simulink model "FM_Bistatic_Radar_Full"  (R2025a)
settings: Solver=VariableStepAuto  StartTime=0.0  StopTime=10.0  RelTol=1e-3
libraries: dspadpt3 x1, commanabbnd3 x1
(part 1 of 3)
settings Model: Creator=leifefrancisco  LastModifiedBy=leifefrancisco

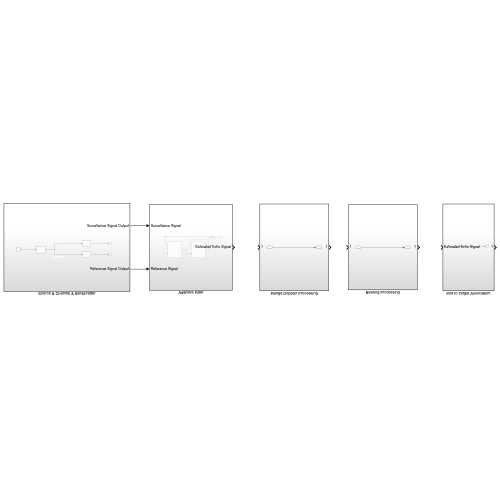
[thumbnail: Simulink's stored preview of the top-level diagram]
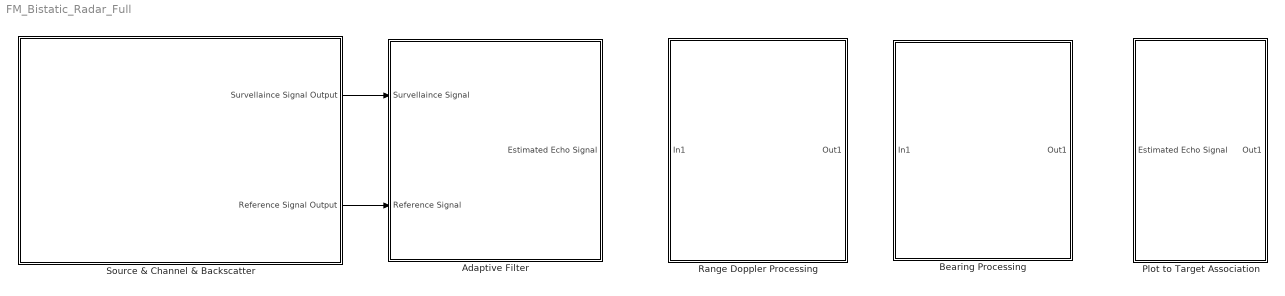
== system FM_Bistatic_Radar_Full ==
  Adaptive Filter : Subsystem
  Bearing Processing : Subsystem
  Plot to Target Association : Subsystem
  Range Doppler Processing : Subsystem
  Source & Channel & Backscatter : Subsystem
  wires:
  Source & Channel & Backscatter/1(Survellaince Signal Output) -> Adaptive Filter/1(Survellaince Signal)
  Source & Channel & Backscatter/2(Reference Signal Output) -> Adaptive Filter/2(Reference Signal)

== system FM_Bistatic_Radar_Full/Adaptive Filter ==
  Survellaince Signal : Inport
  Reference Signal : Inport  Port=2
  Gradiant Adaptive Lattice : Subsystem
  Subtract : Sum  Inputs=+-
  Tapped Delay Line : Subsystem
  Estimated Echo Signal : Outport
  wires:
  Reference Signal/1 -> Gradiant Adaptive Lattice/2(Backwards Propogation Error)
  Survellaince Signal/1 -> Gradiant Adaptive Lattice/1(Forward Propogation Error), Subtract/1
  Gradiant Adaptive Lattice/1(Backards Propogation Error Output) -> Tapped Delay Line/2(Backwards Propogation Errors)
  Tapped Delay Line/1(Error Signal) -> Subtract/2
  Subtract/1 -> Tapped Delay Line/1(Estimated Echo Signal), Estimated Echo Signal/1

== system FM_Bistatic_Radar_Full/Bearing Processing ==
  In1 : Inport
  Out1 : Outport
  wires:
  In1/1 -> Out1/1

== system FM_Bistatic_Radar_Full/Plot to Target Association ==
  Estimated Echo Signal : Inport
  Out1 : Outport
  wires:
  Estimated Echo Signal/1 -> Out1/1

== system FM_Bistatic_Radar_Full/Range Doppler Processing ==
  In1 : Inport
  Out1 : Outport
  wires:
  In1/1 -> Out1/1

== system FM_Bistatic_Radar_Full/Source & Channel & Backscatter ==
  note: Put that function that you made in your matlab code
  note: Survellaince Signal
  note: Reference Signal
  FM Modulator Baseband : commanabbnd3/FM Modulator Baseband  FrequencyDeviation=75e3  SimulateUsing=Code generation
  MATLAB Function : MATLAB Function  TreatAsAtomicUnit=on
  MATLAB Function1 : MATLAB Function  TreatAsAtomicUnit=on
  Sine Wave : Sin  Frequency=2*pi*200*1000  SampleTime=1/10000
  Survellaince Signal Output : Outport
  Reference Signal Output : Outport  Port=2
  wires:
  MATLAB Function/1(y) -> Survellaince Signal Output/1
  MATLAB Function1/1(y) -> Reference Signal Output/1
  Sine Wave/1 -> FM Modulator Baseband/1
  FM Modulator Baseband/1 -> MATLAB Function1/1(u), MATLAB Function/1(u)

== system FM_Bistatic_Radar_Full/Adaptive Filter/Gradiant Adaptive Lattice ==
  Forward Propogation Error : Inport
  Backwards Propogation Error : Inport  Port=2
  50-Stage Lattice Predictor : Subsystem
  Sum of Elements : Sum  Inputs=++++++++++
  Backards Propogation Error Output : Outport
  wires:
  Forward Propogation Error/1 -> 50-Stage Lattice Predictor/1(Forward Prediction Error)
  Backwards Propogation Error/1 -> 50-Stage Lattice Predictor/2(Backward Prediction Error)
  50-Stage Lattice Predictor/1(Backwards Propogation Error1) -> Sum of Elements/1
  50-Stage Lattice Predictor/2(Backwards Propogation Error2) -> Sum of Elements/2
  50-Stage Lattice Predictor/3(Backwards Propogation Error3) -> Sum of Elements/3
  50-Stage Lattice Predictor/4(Backwards Propogation Error4) -> Sum of Elements/4
  50-Stage Lattice Predictor/5(Backwards Propogation Error5) -> Sum of Elements/5
  50-Stage Lattice Predictor/6(Backwards Propogation Error6) -> Sum of Elements/6
  50-Stage Lattice Predictor/7(Backwards Propogation Error7) -> Sum of Elements/7
  50-Stage Lattice Predictor/8(Backwards Propogation Error8) -> Sum of Elements/8
  50-Stage Lattice Predictor/9(Backwards Propogation Error9) -> Sum of Elements/9
  50-Stage Lattice Predictor/10(Backwards Propogation Error10) -> Sum of Elements/10
  Sum of Elements/1 -> Backards Propogation Error Output/1

== system FM_Bistatic_Radar_Full/Adaptive Filter/Tapped Delay Line ==
  Estimated Echo Signal : Inport
  Backwards Propogation Errors : Inport  Port=2
  LMS Filter : dspadpt3/LMS Filter  Algo=LMS  L=32  stepflag=Dialog  mu=0.1  leakage=1.0  ic=0  Adapt=off  resetflag=None  weights=on  addnparflag=off  roundingMode=Floor  overflowMode=off  secondCoeffMode=Binary point scaling  secondCoeffWordLength=2  secondCoeffFracLength=15  prodOutput2Mode=Binary point scaling  prodOutput2FracLength=20  prodOutput3Mode=Binary point scaling  prodOutput3FracLength=20  prodOutput4Mode=Binary point scaling  prodOutput4FracLength=20  quotientMode=Binary point scaling  quotientFracLength=20  accum2Mode=Binary point scaling  accum2FracLength=20
      settings: LibrarySourceBlock=dsphdlsupportfiltering/LMS Filter
  Scope : Scope
  Scope1 : Scope
  Error Signal : Outport
  wires:
  Estimated Echo Signal/1 -> LMS Filter/1
  Backwards Propogation Errors/1 -> LMS Filter/2
  LMS Filter/2 -> Error Signal/1
  LMS Filter/1 -> Scope/1
  LMS Filter/3 -> Scope1/1

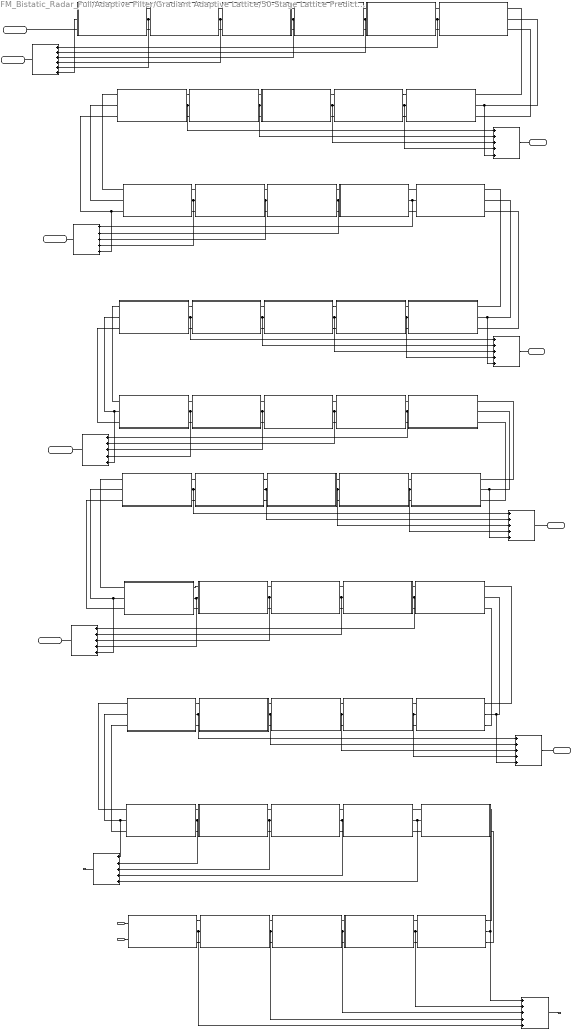
== system FM_Bistatic_Radar_Full/Adaptive Filter/Gradiant Adaptive Lattice/50-Stage Lattice Predictor ==
  Forward Prediction Error : Inport
  Backward Prediction Error : Inport  Port=2
  Stage 1 : Subsystem
  Stage 10 : Subsystem
  Stage 11 : Subsystem
  Stage 12 : Subsystem
  Stage 13 : Subsystem
  Stage 14 : Subsystem
  Stage 15 : Subsystem
  Stage 16 : Subsystem
  Stage 17 : Subsystem
  Stage 18 : Subsystem
  Stage 19 : Subsystem
  Stage 2 : Subsystem
  Stage 20 : Subsystem
  Stage 21 : Subsystem
  Stage 22 : Subsystem
  Stage 23 : Subsystem
  Stage 24 : Subsystem
  Stage 25 : Subsystem
  Stage 26 : Subsystem
  Stage 27 : Subsystem
  Stage 28 : Subsystem
  Stage 29 : Subsystem
  Stage 3 : Subsystem
  Stage 30 : Subsystem
  Stage 31 : Subsystem
  Stage 32 : Subsystem
  Stage 33 : Subsystem
  Stage 34 : Subsystem
  Stage 35 : Subsystem
  Stage 36 : Subsystem
  Stage 37 : Subsystem
  Stage 38 : Subsystem
  Stage 39 : Subsystem
  Stage 4 : Subsystem
  Stage 40 : Subsystem
  Stage 41 : Subsystem
  Stage 42 : Subsystem
  Stage 43 : Subsystem
  Stage 44 : Subsystem
  Stage 45 : Subsystem
  Stage 46 : Subsystem
  Stage 47 : Subsystem
  Stage 48 : Subsystem
  Stage 49 : Subsystem
  Stage 5 : Subsystem
  Stage 50 : Subsystem
  Stage 51 : Subsystem
  Stage 6 : Subsystem
  Stage 7 : Subsystem
  Stage 8 : Subsystem
  Stage 9 : Subsystem
  Sum of Elements{1..9} (9 alike) : Sum  Inputs=+++++
  Sum of Elements10 : Sum  Inputs=++++++
  Backwards Propogation Error1 : Outport
  Backwards Propogation Error2 : Outport  Port=2
  Backwards Propogation Error3 : Outport  Port=3
  Backwards Propogation Error4 : Outport  Port=4
  Backwards Propogation Error5 : Outport  Port=5
  Backwards Propogation Error6 : Outport  Port=6
  Backwards Propogation Error7 : Outport  Port=7
  Backwards Propogation Error8 : Outport  Port=8
  Backwards Propogation Error9 : Outport  Port=9
  Backwards Propogation Error10 : Outport  Port=10
  K Final : Outport  Port=11
  wires:
  Stage 9/2(Backward Prediction Error Output) -> Sum of Elements2/2, Stage 10/2(Backward Prediction Error)
  Backward Prediction Error/1 -> Stage 1/2(Backward Prediction Error)
  Stage 50/1(Forward Prediction Error Output) -> Stage 51/1(Forward Prediction Error)
  Stage 29/3(K) -> Stage 30/3(K Input)
  Stage 21/3(K) -> Stage 22/3(K Input)
  Stage 36/3(K) -> Stage 37/3(K Input)
  Stage 27/3(K) -> Stage 28/3(K Input)
  Stage 15/3(K) -> Stage 16/3(K Input)
  Stage 20/3(K) -> Stage 21/3(K Input)
  Stage 49/1(Forward Prediction Error Output) -> Stage 50/1(Forward Prediction Error)
  Stage 47/3(K) -> Stage 48/3(K Input)
  Stage 20/2(Backward Prediction Error Output) -> Sum of Elements6/3, Stage 21/2(Backward Prediction Error)
  Stage 46/1(Forward Prediction Error Output) -> Stage 47/1(Forward Prediction Error)
  Stage 18/1(Forward Prediction Error Output) -> Stage 19/1(Forward Prediction Error)
  Stage 5/3(K) -> Stage 6/3(K Input)
  Stage 46/3(K) -> Stage 47/3(K Input)
  Stage 17/2(Backward Prediction Error Output) -> Sum of Elements4/2, Stage 26/2(Backward Prediction Error)
  Stage 50/2(Backward Prediction Error Output) -> Sum of Elements10/5, Stage 51/2(Backward Prediction Error)
  Stage 25/3(K) -> Stage 34/3(K Input)
  Forward Prediction Error/1 -> Stage 1/1(Forward Prediction Error)
  Stage 38/3(K) -> Stage 39/3(K Input)
  Stage 11/2(Backward Prediction Error Output) -> Sum of Elements3/1, Stage 12/2(Backward Prediction Error)
  Stage 2/3(K) -> Stage 3/3(K Input)
  Stage 24/2(Backward Prediction Error Output) -> Sum of Elements7/2, Stage 25/2(Backward Prediction Error)
  Stage 7/2(Backward Prediction Error Output) -> Sum of Elements2/4, Stage 8/2(Backward Prediction Error)
  Stage 18/2(Backward Prediction Error Output) -> Sum of Elements6/1, Stage 19/2(Backward Prediction Error)
  Stage 37/2(Backward Prediction Error Output) -> Sum of Elements8/2, Stage 38/2(Backward Prediction Error)
  Stage 32/2(Backward Prediction Error Output) -> Sum of Elements5/4, Stage 33/2(Backward Prediction Error)
  Stage 48/2(Backward Prediction Error Output) -> Sum of Elements10/3, Stage 49/2(Backward Prediction Error)
  Stage 49/3(K) -> Stage 50/3(K Input)
  Stage 30/1(Forward Prediction Error Output) -> Stage 31/1(Forward Prediction Error)
  Stage 21/2(Backward Prediction Error Output) -> Sum of Elements6/4, Stage 22/2(Backward Prediction Error)
  Stage 38/1(Forward Prediction Error Output) -> Stage 39/1(Forward Prediction Error)
  Stage 39/2(Backward Prediction Error Output) -> Sum of Elements8/4, Stage 40/2(Backward Prediction Error)
  Stage 21/1(Forward Prediction Error Output) -> Stage 22/1(Forward Prediction Error)
  Stage 36/2(Backward Prediction Error Output) -> Sum of Elements8/1, Stage 37/2(Backward Prediction Error)
  Stage 34/3(K) -> Stage 35/3(K Input)
  Stage 29/1(Forward Prediction Error Output) -> Stage 30/1(Forward Prediction Error)
  Stage 48/1(Forward Prediction Error Output) -> Stage 49/1(Forward Prediction Error)
  Stage 39/3(K) -> Stage 40/3(K Input)
  Stage 3/3(K) -> Stage 4/3(K Input)
  Stage 14/3(K) -> Stage 15/3(K Input)
  Stage 25/1(Forward Prediction Error Output) -> Stage 34/1(Forward Prediction Error)
  Stage 19/3(K) -> Stage 20/3(K Input)
  Stage 24/1(Forward Prediction Error Output) -> Stage 25/1(Forward Prediction Error)
  Stage 9/1(Forward Prediction Error Output) -> Stage 10/1(Forward Prediction Error)
  Stage 24/3(K) -> Stage 25/3(K Input)
  Stage 17/3(K) -> Stage 26/3(K Input)
  Stage 29/2(Backward Prediction Error Output) -> Sum of Elements5/1, Stage 30/2(Backward Prediction Error)
  Stage 7/1(Forward Prediction Error Output) -> Stage 8/1(Forward Prediction Error)
  Stage 34/2(Backward Prediction Error Output) -> Sum of Elements7/4, Stage 35/2(Backward Prediction Error)
  Stage 19/1(Forward Prediction Error Output) -> Stage 20/1(Forward Prediction Error)
  Stage 1/1(Forward Prediction Error Output) -> Stage 2/1(Forward Prediction Error)
  Stage 23/3(K) -> Stage 24/3(K Input)
  Stage 23/2(Backward Prediction Error Output) -> Sum of Elements7/1, Stage 24/2(Backward Prediction Error)
  Stage 37/3(K) -> Stage 38/3(K Input)
  Stage 20/1(Forward Prediction Error Output) -> Stage 21/1(Forward Prediction Error)
  Stage 19/2(Backward Prediction Error Output) -> Sum of Elements6/2, Stage 20/2(Backward Prediction Error)
  Stage 34/1(Forward Prediction Error Output) -> Stage 35/1(Forward Prediction Error)
  Stage 23/1(Forward Prediction Error Output) -> Stage 24/1(Forward Prediction Error)
  Stage 6/1(Forward Prediction Error Output) -> Stage 7/1(Forward Prediction Error)
  Stage 4/3(K) -> Stage 5/3(K Input)
  Stage 12/1(Forward Prediction Error Output) -> Stage 13/1(Forward Prediction Error)
  Stage 32/1(Forward Prediction Error Output) -> Stage 33/1(Forward Prediction Error)
  Stage 32/3(K) -> Stage 33/3(K Input)
  Stage 39/1(Forward Prediction Error Output) -> Stage 40/1(Forward Prediction Error)
  Stage 1/3(K) -> Stage 2/3(K Input)
  Stage 8/1(Forward Prediction Error Output) -> Stage 9/1(Forward Prediction Error)
  Stage 26/2(Backward Prediction Error Output) -> Sum of Elements4/3, Stage 27/2(Backward Prediction Error)
  Stage 27/2(Backward Prediction Error Output) -> Sum of Elements4/4, Stage 28/2(Backward Prediction Error)
  Stage 25/2(Backward Prediction Error Output) -> Sum of Elements7/3, Stage 34/2(Backward Prediction Error)
  Stage 6/3(K) -> Stage 7/3(K Input)
  Stage 27/1(Forward Prediction Error Output) -> Stage 28/1(Forward Prediction Error)
  Stage 30/3(K) -> Stage 31/3(K Input)
  Stage 3/2(Backward Prediction Error Output) -> Sum of Elements1/3, Stage 4/2(Backward Prediction Error)
  Stage 31/3(K) -> Stage 32/3(K Input)
  Stage 47/1(Forward Prediction Error Output) -> Stage 48/1(Forward Prediction Error)
  Stage 49/2(Backward Prediction Error Output) -> Sum of Elements10/4, Stage 50/2(Backward Prediction Error)
  Stage 46/2(Backward Prediction Error Output) -> Sum of Elements10/1, Stage 47/2(Backward Prediction Error)
  Stage 26/3(K) -> Stage 27/3(K Input)
  Stage 11/1(Forward Prediction Error Output) -> Stage 12/1(Forward Prediction Error)
  Stage 31/2(Backward Prediction Error Output) -> Sum of Elements5/3, Stage 32/2(Backward Prediction Error)
  Stage 50/3(K) -> Stage 51/3(K Input)
  Stage 31/1(Forward Prediction Error Output) -> Stage 32/1(Forward Prediction Error)
  Stage 26/1(Forward Prediction Error Output) -> Stage 27/1(Forward Prediction Error)
  Stage 48/3(K) -> Stage 49/3(K Input)
  Stage 37/1(Forward Prediction Error Output) -> Stage 38/1(Forward Prediction Error)
  Stage 4/2(Backward Prediction Error Output) -> Sum of Elements1/2, Stage 5/2(Backward Prediction Error)
  Stage 2/1(Forward Prediction Error Output) -> Stage 3/1(Forward Prediction Error)
  Stage 17/1(Forward Prediction Error Output) -> Stage 26/1(Forward Prediction Error)
  Stage 16/2(Backward Prediction Error Output) -> Sum of Elements4/1, Stage 17/2(Backward Prediction Error)
  Stage 15/2(Backward Prediction Error Output) -> Sum of Elements3/5, Stage 16/2(Backward Prediction Error)
  Stage 18/3(K) -> Stage 19/3(K Input)
  Stage 14/1(Forward Prediction Error Output) -> Stage 15/1(Forward Prediction Error)
  Stage 12/2(Backward Prediction Error Output) -> Sum of Elements3/2, Stage 13/2(Backward Prediction Error)
  Stage 38/2(Backward Prediction Error Output) -> Sum of Elements8/3, Stage 39/2(Backward Prediction Error)
  Stage 8/2(Backward Prediction Error Output) -> Sum of Elements2/3, Stage 9/2(Backward Prediction Error)
  Stage 13/1(Forward Prediction Error Output) -> Stage 14/1(Forward Prediction Error)
  Stage 16/1(Forward Prediction Error Output) -> Stage 17/1(Forward Prediction Error)
  Stage 5/1(Forward Prediction Error Output) -> Stage 6/1(Forward Prediction Error)
  Stage 14/2(Backward Prediction Error Output) -> Sum of Elements3/4, Stage 15/2(Backward Prediction Error)
  Stage 6/2(Backward Prediction Error Output) -> Sum of Elements2/5, Stage 7/2(Backward Prediction Error)
  Stage 12/3(K) -> Stage 13/3(K Input)
  Stage 16/3(K) -> Stage 17/3(K Input)
  Stage 15/1(Forward Prediction Error Output) -> Stage 16/1(Forward Prediction Error)
  Stage 13/2(Backward Prediction Error Output) -> Sum of Elements3/3, Stage 14/2(Backward Prediction Error)
  Stage 11/3(K) -> Stage 12/3(K Input)
  Stage 4/1(Forward Prediction Error Output) -> Stage 5/1(Forward Prediction Error)
  Stage 5/2(Backward Prediction Error Output) -> Sum of Elements1/1, Stage 6/2(Backward Prediction Error)
  Stage 9/3(K) -> Stage 10/3(K Input)
  Stage 8/3(K) -> Stage 9/3(K Input)
  Stage 13/3(K) -> Stage 14/3(K Input)
  Stage 7/3(K) -> Stage 8/3(K Input)
  Stage 36/1(Forward Prediction Error Output) -> Stage 37/1(Forward Prediction Error)
  Stage 3/1(Forward Prediction Error Output) -> Stage 4/1(Forward Prediction Error)
  Stage 47/2(Backward Prediction Error Output) -> Sum of Elements10/2, Stage 48/2(Backward Prediction Error)
  Stage 30/2(Backward Prediction Error Output) -> Sum of Elements5/2, Stage 31/2(Backward Prediction Error)
  Stage 1/2(Backward Prediction Error Output) -> Sum of Elements1/5, Stage 2/2(Backward Prediction Error)
  Stage 10/3(K) -> Stage 11/3(K Input)
  Stage 10/2(Backward Prediction Error Output) -> Sum of Elements2/1, Stage 11/2(Backward Prediction Error)
  Stage 10/1(Forward Prediction Error Output) -> Stage 11/1(Forward Prediction Error)
  Stage 28/3(K) -> Stage 29/3(K Input)
  Stage 28/2(Backward Prediction Error Output) -> Sum of Elements4/5, Stage 29/2(Backward Prediction Error)
  Stage 28/1(Forward Prediction Error Output) -> Stage 29/1(Forward Prediction Error)
  Stage 33/3(K) -> Stage 18/3(K Input)
  Stage 33/2(Backward Prediction Error Output) -> Sum of Elements5/5, Stage 18/2(Backward Prediction Error)
  Stage 33/1(Forward Prediction Error Output) -> Stage 18/1(Forward Prediction Error)
  Stage 22/3(K) -> Stage 23/3(K Input)
  Stage 22/2(Backward Prediction Error Output) -> Sum of Elements6/5, Stage 23/2(Backward Prediction Error)
  Stage 22/1(Forward Prediction Error Output) -> Stage 23/1(Forward Prediction Error)
  Stage 35/3(K) -> Stage 36/3(K Input)
  Stage 35/2(Backward Prediction Error Output) -> Sum of Elements7/5, Stage 36/2(Backward Prediction Error)
  Stage 35/1(Forward Prediction Error Output) -> Stage 36/1(Forward Prediction Error)
  Stage 40/2(Backward Prediction Error Output) -> Stage 41/2(Backward Prediction Error)
  Stage 40/1(Forward Prediction Error Output) -> Stage 41/1(Forward Prediction Error)
  Stage 41/1(Forward Prediction Error Output) -> Stage 42/1(Forward Prediction Error)
  Stage 41/2(Backward Prediction Error Output) -> Sum of Elements9/1, Stage 42/2(Backward Prediction Error)
  Stage 41/3(K) -> Stage 42/3(K Input)
  Stage 42/1(Forward Prediction Error Output) -> Stage 43/1(Forward Prediction Error)
  Stage 42/2(Backward Prediction Error Output) -> Sum of Elements9/2, Stage 43/2(Backward Prediction Error)
  Stage 42/3(K) -> Stage 43/3(K Input)
  Stage 43/1(Forward Prediction Error Output) -> Stage 44/1(Forward Prediction Error)
  Stage 43/2(Backward Prediction Error Output) -> Sum of Elements9/3, Stage 44/2(Backward Prediction Error)
  Stage 43/3(K) -> Stage 44/3(K Input)
  Stage 44/1(Forward Prediction Error Output) -> Stage 45/1(Forward Prediction Error)
  Stage 44/2(Backward Prediction Error Output) -> Sum of Elements9/4, Stage 45/2(Backward Prediction Error)
  Stage 44/3(K) -> Stage 45/3(K Input)
  Stage 45/3(K) -> Stage 46/3(K Input)
  Stage 45/2(Backward Prediction Error Output) -> Sum of Elements9/5, Stage 46/2(Backward Prediction Error)
  Stage 45/1(Forward Prediction Error Output) -> Stage 46/1(Forward Prediction Error)
  Stage 40/3(K) -> Stage 41/3(K Input), Sum of Elements8/5
  Stage 2/2(Backward Prediction Error Output) -> Sum of Elements1/4, Stage 3/2(Backward Prediction Error)
  Sum of Elements1/1 -> Backwards Propogation Error1/1
  Sum of Elements2/1 -> Backwards Propogation Error2/1
  Stage 51/2(Backward Prediction Error Output) -> Sum of Elements10/6
  Sum of Elements10/1 -> Backwards Propogation Error10/1
  Sum of Elements8/1 -> Backwards Propogation Error8/1
  Sum of Elements6/1 -> Backwards Propogation Error6/1
  Sum of Elements4/1 -> Backwards Propogation Error4/1
  Sum of Elements3/1 -> Backwards Propogation Error3/1
  Sum of Elements5/1 -> Backwards Propogation Error5/1
  Sum of Elements7/1 -> Backwards Propogation Error7/1
  Sum of Elements9/1 -> Backwards Propogation Error9/1
  Stage 51/3(K) -> K Final/1

== system FM_Bistatic_Radar_Full/Adaptive Filter/Gradiant Adaptive Lattice/50-Stage Lattice Predictor/Stage 1 ==
  note: K Update
  Forward Prediction Error : Inport
  Backward Prediction Error : Inport  Port=2
  Delay : Delay  DelayLength=1  InitialCondition=0
  K Update Equation : Subsystem
  Sum : Sum  Inputs=|++
  Sum1 : Sum  Inputs=|++
  Forward Prediction Error Output : Outport
  Backward Prediction Error Output : Outport  Port=2
  K : Outport  Port=3
  wires:
  Sum1/1 -> Backward Prediction Error Output/1
  Delay/1 -> Sum1/2, K Update Equation/2(B I/P)
  Sum/1 -> Forward Prediction Error Output/1
  K Update Equation/2(K) -> K/1, Sum1/1
  K Update Equation/1(*K (K conjugate)) -> Sum/2
  Backward Prediction Error/1 -> Delay/1
  Forward Prediction Error/1 -> Sum/1, K Update Equation/1(F I/P)

== system FM_Bistatic_Radar_Full/Adaptive Filter/Gradiant Adaptive Lattice/50-Stage Lattice Predictor/Stage 10 ==
  note: K Update
  Forward Prediction Error : Inport
  Backward Prediction Error : Inport  Port=2
  K Input : Inport  Port=3
  Delay : Delay  DelayLength=1  InitialCondition=0
  K Update Equation : Subsystem
  Sum : Sum  Inputs=|++
  Sum1 : Sum  Inputs=|++
  Forward Prediction Error Output : Outport
  Backward Prediction Error Output : Outport  Port=2
  K : Outport  Port=3
  wires:
  Sum1/1 -> Backward Prediction Error Output/1
  Delay/1 -> Sum1/2, K Update Equation/2(B I/P)
  Sum/1 -> Forward Prediction Error Output/1
  K Update Equation/2(K) -> K/1, Sum1/1
  K Update Equation/1(*K (K conjugate)) -> Sum/2
  Backward Prediction Error/1 -> Delay/1
  Forward Prediction Error/1 -> Sum/1, K Update Equation/1(F I/P)
  K Input/1 -> K Update Equation/3(K I/P)

== system FM_Bistatic_Radar_Full/Adaptive Filter/Gradiant Adaptive Lattice/50-Stage Lattice Predictor/Stage 11 ==
  note: K Update
  Forward Prediction Error : Inport
  Backward Prediction Error : Inport  Port=2
  K Input : Inport  Port=3
  Delay : Delay  DelayLength=1  InitialCondition=0
  K Update Equation : Subsystem
  Sum : Sum  Inputs=|++
  Sum1 : Sum  Inputs=|++
  Forward Prediction Error Output : Outport
  Backward Prediction Error Output : Outport  Port=2
  K : Outport  Port=3
  wires:
  Sum1/1 -> Backward Prediction Error Output/1
  Delay/1 -> Sum1/2, K Update Equation/2(B I/P)
  Sum/1 -> Forward Prediction Error Output/1
  K Update Equation/2(K) -> K/1, Sum1/1
  K Update Equation/1(*K (K conjugate)) -> Sum/2
  Backward Prediction Error/1 -> Delay/1
  Forward Prediction Error/1 -> Sum/1, K Update Equation/1(F I/P)
  K Input/1 -> K Update Equation/3(K I/P)

== system FM_Bistatic_Radar_Full/Adaptive Filter/Gradiant Adaptive Lattice/50-Stage Lattice Predictor/Stage 12 ==
  note: K Update
  Forward Prediction Error : Inport
  Backward Prediction Error : Inport  Port=2
  K Input : Inport  Port=3
  Delay : Delay  DelayLength=1  InitialCondition=0
  K Update Equation : Subsystem
  Sum : Sum  Inputs=|++
  Sum1 : Sum  Inputs=|++
  Forward Prediction Error Output : Outport
  Backward Prediction Error Output : Outport  Port=2
  K : Outport  Port=3
  wires:
  Sum1/1 -> Backward Prediction Error Output/1
  Delay/1 -> Sum1/2, K Update Equation/2(B I/P)
  Sum/1 -> Forward Prediction Error Output/1
  K Update Equation/2(K) -> K/1, Sum1/1
  K Update Equation/1(*K (K conjugate)) -> Sum/2
  Backward Prediction Error/1 -> Delay/1
  Forward Prediction Error/1 -> Sum/1, K Update Equation/1(F I/P)
  K Input/1 -> K Update Equation/3(K I/P)

== system FM_Bistatic_Radar_Full/Adaptive Filter/Gradiant Adaptive Lattice/50-Stage Lattice Predictor/Stage 13 ==
  note: K Update
  Forward Prediction Error : Inport
  Backward Prediction Error : Inport  Port=2
  K Input : Inport  Port=3
  Delay : Delay  DelayLength=1  InitialCondition=0
  K Update Equation : Subsystem
  Sum : Sum  Inputs=|++
  Sum1 : Sum  Inputs=|++
  Forward Prediction Error Output : Outport
  Backward Prediction Error Output : Outport  Port=2
  K : Outport  Port=3
  wires:
  Sum1/1 -> Backward Prediction Error Output/1
  Delay/1 -> Sum1/2, K Update Equation/2(B I/P)
  Sum/1 -> Forward Prediction Error Output/1
  K Update Equation/2(K) -> K/1, Sum1/1
  K Update Equation/1(*K (K conjugate)) -> Sum/2
  Backward Prediction Error/1 -> Delay/1
  Forward Prediction Error/1 -> Sum/1, K Update Equation/1(F I/P)
  K Input/1 -> K Update Equation/3(K I/P)

== system FM_Bistatic_Radar_Full/Adaptive Filter/Gradiant Adaptive Lattice/50-Stage Lattice Predictor/Stage 14 ==
  note: K Update
  Forward Prediction Error : Inport
  Backward Prediction Error : Inport  Port=2
  K Input : Inport  Port=3
  Delay : Delay  DelayLength=1  InitialCondition=0
  K Update Equation : Subsystem
  Sum : Sum  Inputs=|++
  Sum1 : Sum  Inputs=|++
  Forward Prediction Error Output : Outport
  Backward Prediction Error Output : Outport  Port=2
  K : Outport  Port=3
  wires:
  Sum1/1 -> Backward Prediction Error Output/1
  Delay/1 -> Sum1/2, K Update Equation/2(B I/P)
  Sum/1 -> Forward Prediction Error Output/1
  K Update Equation/2(K) -> K/1, Sum1/1
  K Update Equation/1(*K (K conjugate)) -> Sum/2
  Backward Prediction Error/1 -> Delay/1
  Forward Prediction Error/1 -> Sum/1, K Update Equation/1(F I/P)
  K Input/1 -> K Update Equation/3(K I/P)

== system FM_Bistatic_Radar_Full/Adaptive Filter/Gradiant Adaptive Lattice/50-Stage Lattice Predictor/Stage 15 ==
  note: K Update
  Forward Prediction Error : Inport
  Backward Prediction Error : Inport  Port=2
  K Input : Inport  Port=3
  Delay : Delay  DelayLength=1  InitialCondition=0
  K Update Equation : Subsystem
  Sum : Sum  Inputs=|++
  Sum1 : Sum  Inputs=|++
  Forward Prediction Error Output : Outport
  Backward Prediction Error Output : Outport  Port=2
  K : Outport  Port=3
  wires:
  Sum1/1 -> Backward Prediction Error Output/1
  Delay/1 -> Sum1/2, K Update Equation/2(B I/P)
  Sum/1 -> Forward Prediction Error Output/1
  K Update Equation/2(K) -> K/1, Sum1/1
  K Update Equation/1(*K (K conjugate)) -> Sum/2
  Backward Prediction Error/1 -> Delay/1
  Forward Prediction Error/1 -> Sum/1, K Update Equation/1(F I/P)
  K Input/1 -> K Update Equation/3(K I/P)

== system FM_Bistatic_Radar_Full/Adaptive Filter/Gradiant Adaptive Lattice/50-Stage Lattice Predictor/Stage 16 ==
  note: K Update
  Forward Prediction Error : Inport
  Backward Prediction Error : Inport  Port=2
  K Input : Inport  Port=3
  Delay : Delay  DelayLength=1  InitialCondition=0
  K Update Equation : Subsystem
  Sum : Sum  Inputs=|++
  Sum1 : Sum  Inputs=|++
  Forward Prediction Error Output : Outport
  Backward Prediction Error Output : Outport  Port=2
  K : Outport  Port=3
  wires:
  Sum1/1 -> Backward Prediction Error Output/1
  Delay/1 -> Sum1/2, K Update Equation/2(B I/P)
  Sum/1 -> Forward Prediction Error Output/1
  K Update Equation/2(K) -> K/1, Sum1/1
  K Update Equation/1(*K (K conjugate)) -> Sum/2
  Backward Prediction Error/1 -> Delay/1
  Forward Prediction Error/1 -> Sum/1, K Update Equation/1(F I/P)
  K Input/1 -> K Update Equation/3(K I/P)

== system FM_Bistatic_Radar_Full/Adaptive Filter/Gradiant Adaptive Lattice/50-Stage Lattice Predictor/Stage 17 ==
  note: K Update
  Forward Prediction Error : Inport
  Backward Prediction Error : Inport  Port=2
  K Input : Inport  Port=3
  Delay : Delay  DelayLength=1  InitialCondition=0
  K Update Equation : Subsystem
  Sum : Sum  Inputs=|++
  Sum1 : Sum  Inputs=|++
  Forward Prediction Error Output : Outport
  Backward Prediction Error Output : Outport  Port=2
  K : Outport  Port=3
  wires:
  Sum1/1 -> Backward Prediction Error Output/1
  Delay/1 -> Sum1/2, K Update Equation/2(B I/P)
  Sum/1 -> Forward Prediction Error Output/1
  K Update Equation/2(K) -> K/1, Sum1/1
  K Update Equation/1(*K (K conjugate)) -> Sum/2
  Backward Prediction Error/1 -> Delay/1
  Forward Prediction Error/1 -> Sum/1, K Update Equation/1(F I/P)
  K Input/1 -> K Update Equation/3(K I/P)

== system FM_Bistatic_Radar_Full/Adaptive Filter/Gradiant Adaptive Lattice/50-Stage Lattice Predictor/Stage 18 ==
  note: K Update
  Forward Prediction Error : Inport
  Backward Prediction Error : Inport  Port=2
  K Input : Inport  Port=3
  Delay : Delay  DelayLength=1  InitialCondition=0
  K Update Equation : Subsystem
  Sum : Sum  Inputs=|++
  Sum1 : Sum  Inputs=|++
  Forward Prediction Error Output : Outport
  Backward Prediction Error Output : Outport  Port=2
  K : Outport  Port=3
  wires:
  Sum1/1 -> Backward Prediction Error Output/1
  Delay/1 -> Sum1/2, K Update Equation/2(B I/P)
  Sum/1 -> Forward Prediction Error Output/1
  K Update Equation/2(K) -> K/1, Sum1/1
  K Update Equation/1(*K (K conjugate)) -> Sum/2
  Backward Prediction Error/1 -> Delay/1
  Forward Prediction Error/1 -> Sum/1, K Update Equation/1(F I/P)
  K Input/1 -> K Update Equation/3(K I/P)

== system FM_Bistatic_Radar_Full/Adaptive Filter/Gradiant Adaptive Lattice/50-Stage Lattice Predictor/Stage 19 ==
  note: K Update
  Forward Prediction Error : Inport
  Backward Prediction Error : Inport  Port=2
  K Input : Inport  Port=3
  Delay : Delay  DelayLength=1  InitialCondition=0
  K Update Equation : Subsystem
  Sum : Sum  Inputs=|++
  Sum1 : Sum  Inputs=|++
  Forward Prediction Error Output : Outport
  Backward Prediction Error Output : Outport  Port=2
  K : Outport  Port=3
  wires:
  Sum1/1 -> Backward Prediction Error Output/1
  Delay/1 -> Sum1/2, K Update Equation/2(B I/P)
  Sum/1 -> Forward Prediction Error Output/1
  K Update Equation/2(K) -> K/1, Sum1/1
  K Update Equation/1(*K (K conjugate)) -> Sum/2
  Backward Prediction Error/1 -> Delay/1
  Forward Prediction Error/1 -> Sum/1, K Update Equation/1(F I/P)
  K Input/1 -> K Update Equation/3(K I/P)

== system FM_Bistatic_Radar_Full/Adaptive Filter/Gradiant Adaptive Lattice/50-Stage Lattice Predictor/Stage 2 ==
  note: K Update
  Forward Prediction Error : Inport
  Backward Prediction Error : Inport  Port=2
  K Input : Inport  Port=3
  Delay : Delay  DelayLength=1  InitialCondition=0
  K Update Equation : Subsystem
  Sum : Sum  Inputs=|++
  Sum1 : Sum  Inputs=|++
  Forward Prediction Error Output : Outport
  Backward Prediction Error Output : Outport  Port=2
  K : Outport  Port=3
  wires:
  Sum1/1 -> Backward Prediction Error Output/1
  Delay/1 -> Sum1/2, K Update Equation/2(B I/P)
  Sum/1 -> Forward Prediction Error Output/1
  K Update Equation/2(K) -> K/1, Sum1/1
  K Update Equation/1(*K (K conjugate)) -> Sum/2
  Backward Prediction Error/1 -> Delay/1
  Forward Prediction Error/1 -> Sum/1, K Update Equation/1(F I/P)
  K Input/1 -> K Update Equation/3(K I/P)

== system FM_Bistatic_Radar_Full/Adaptive Filter/Gradiant Adaptive Lattice/50-Stage Lattice Predictor/Stage 20 ==
  note: K Update
  Forward Prediction Error : Inport
  Backward Prediction Error : Inport  Port=2
  K Input : Inport  Port=3
  Delay : Delay  DelayLength=1  InitialCondition=0
  K Update Equation : Subsystem
  Sum : Sum  Inputs=|++
  Sum1 : Sum  Inputs=|++
  Forward Prediction Error Output : Outport
  Backward Prediction Error Output : Outport  Port=2
  K : Outport  Port=3
  wires:
  Sum1/1 -> Backward Prediction Error Output/1
  Delay/1 -> Sum1/2, K Update Equation/2(B I/P)
  Sum/1 -> Forward Prediction Error Output/1
  K Update Equation/2(K) -> K/1, Sum1/1
  K Update Equation/1(*K (K conjugate)) -> Sum/2
  Backward Prediction Error/1 -> Delay/1
  Forward Prediction Error/1 -> Sum/1, K Update Equation/1(F I/P)
  K Input/1 -> K Update Equation/3(K I/P)

== system FM_Bistatic_Radar_Full/Adaptive Filter/Gradiant Adaptive Lattice/50-Stage Lattice Predictor/Stage 21 ==
  note: K Update
  Forward Prediction Error : Inport
  Backward Prediction Error : Inport  Port=2
  K Input : Inport  Port=3
  Delay : Delay  DelayLength=1  InitialCondition=0
  K Update Equation : Subsystem
  Sum : Sum  Inputs=|++
  Sum1 : Sum  Inputs=|++
  Forward Prediction Error Output : Outport
  Backward Prediction Error Output : Outport  Port=2
  K : Outport  Port=3
  wires:
  Sum1/1 -> Backward Prediction Error Output/1
  Delay/1 -> Sum1/2, K Update Equation/2(B I/P)
  Sum/1 -> Forward Prediction Error Output/1
  K Update Equation/2(K) -> K/1, Sum1/1
  K Update Equation/1(*K (K conjugate)) -> Sum/2
  Backward Prediction Error/1 -> Delay/1
  Forward Prediction Error/1 -> Sum/1, K Update Equation/1(F I/P)
  K Input/1 -> K Update Equation/3(K I/P)

== system FM_Bistatic_Radar_Full/Adaptive Filter/Gradiant Adaptive Lattice/50-Stage Lattice Predictor/Stage 22 ==
  note: K Update
  Forward Prediction Error : Inport
  Backward Prediction Error : Inport  Port=2
  K Input : Inport  Port=3
  Delay : Delay  DelayLength=1  InitialCondition=0
  K Update Equation : Subsystem
  Sum : Sum  Inputs=|++
  Sum1 : Sum  Inputs=|++
  Forward Prediction Error Output : Outport
  Backward Prediction Error Output : Outport  Port=2
  K : Outport  Port=3
  wires:
  Sum1/1 -> Backward Prediction Error Output/1
  Delay/1 -> Sum1/2, K Update Equation/2(B I/P)
  Sum/1 -> Forward Prediction Error Output/1
  K Update Equation/2(K) -> K/1, Sum1/1
  K Update Equation/1(*K (K conjugate)) -> Sum/2
  Backward Prediction Error/1 -> Delay/1
  Forward Prediction Error/1 -> Sum/1, K Update Equation/1(F I/P)
  K Input/1 -> K Update Equation/3(K I/P)

== system FM_Bistatic_Radar_Full/Adaptive Filter/Gradiant Adaptive Lattice/50-Stage Lattice Predictor/Stage 23 ==
  note: K Update
  Forward Prediction Error : Inport
  Backward Prediction Error : Inport  Port=2
  K Input : Inport  Port=3
  Delay : Delay  DelayLength=1  InitialCondition=0
  K Update Equation : Subsystem
  Sum : Sum  Inputs=|++
  Sum1 : Sum  Inputs=|++
  Forward Prediction Error Output : Outport
  Backward Prediction Error Output : Outport  Port=2
  K : Outport  Port=3
  wires:
  Sum1/1 -> Backward Prediction Error Output/1
  Delay/1 -> Sum1/2, K Update Equation/2(B I/P)
  Sum/1 -> Forward Prediction Error Output/1
  K Update Equation/2(K) -> K/1, Sum1/1
  K Update Equation/1(*K (K conjugate)) -> Sum/2
  Backward Prediction Error/1 -> Delay/1
  Forward Prediction Error/1 -> Sum/1, K Update Equation/1(F I/P)
  K Input/1 -> K Update Equation/3(K I/P)

== system FM_Bistatic_Radar_Full/Adaptive Filter/Gradiant Adaptive Lattice/50-Stage Lattice Predictor/Stage 24 ==
  note: K Update
  Forward Prediction Error : Inport
  Backward Prediction Error : Inport  Port=2
  K Input : Inport  Port=3
  Delay : Delay  DelayLength=1  InitialCondition=0
  K Update Equation : Subsystem
  Sum : Sum  Inputs=|++
  Sum1 : Sum  Inputs=|++
  Forward Prediction Error Output : Outport
  Backward Prediction Error Output : Outport  Port=2
  K : Outport  Port=3
  wires:
  Sum1/1 -> Backward Prediction Error Output/1
  Delay/1 -> Sum1/2, K Update Equation/2(B I/P)
  Sum/1 -> Forward Prediction Error Output/1
  K Update Equation/2(K) -> K/1, Sum1/1
  K Update Equation/1(*K (K conjugate)) -> Sum/2
  Backward Prediction Error/1 -> Delay/1
  Forward Prediction Error/1 -> Sum/1, K Update Equation/1(F I/P)
  K Input/1 -> K Update Equation/3(K I/P)

== system FM_Bistatic_Radar_Full/Adaptive Filter/Gradiant Adaptive Lattice/50-Stage Lattice Predictor/Stage 25 ==
  note: K Update
  Forward Prediction Error : Inport
  Backward Prediction Error : Inport  Port=2
  K Input : Inport  Port=3
  Delay : Delay  DelayLength=1  InitialCondition=0
  K Update Equation : Subsystem
  Sum : Sum  Inputs=|++
  Sum1 : Sum  Inputs=|++
  Forward Prediction Error Output : Outport
  Backward Prediction Error Output : Outport  Port=2
  K : Outport  Port=3
  wires:
  Sum1/1 -> Backward Prediction Error Output/1
  Delay/1 -> Sum1/2, K Update Equation/2(B I/P)
  Sum/1 -> Forward Prediction Error Output/1
  K Update Equation/2(K) -> K/1, Sum1/1
  K Update Equation/1(*K (K conjugate)) -> Sum/2
  Backward Prediction Error/1 -> Delay/1
  Forward Prediction Error/1 -> Sum/1, K Update Equation/1(F I/P)
  K Input/1 -> K Update Equation/3(K I/P)

== system FM_Bistatic_Radar_Full/Adaptive Filter/Gradiant Adaptive Lattice/50-Stage Lattice Predictor/Stage 26 ==
  note: K Update
  Forward Prediction Error : Inport
  Backward Prediction Error : Inport  Port=2
  K Input : Inport  Port=3
  Delay : Delay  DelayLength=1  InitialCondition=0
  K Update Equation : Subsystem
  Sum : Sum  Inputs=|++
  Sum1 : Sum  Inputs=|++
  Forward Prediction Error Output : Outport
  Backward Prediction Error Output : Outport  Port=2
  K : Outport  Port=3
  wires:
  Sum1/1 -> Backward Prediction Error Output/1
  Delay/1 -> Sum1/2, K Update Equation/2(B I/P)
  Sum/1 -> Forward Prediction Error Output/1
  K Update Equation/2(K) -> K/1, Sum1/1
  K Update Equation/1(*K (K conjugate)) -> Sum/2
  Backward Prediction Error/1 -> Delay/1
  Forward Prediction Error/1 -> Sum/1, K Update Equation/1(F I/P)
  K Input/1 -> K Update Equation/3(K I/P)

== system FM_Bistatic_Radar_Full/Adaptive Filter/Gradiant Adaptive Lattice/50-Stage Lattice Predictor/Stage 27 ==
  note: K Update
  Forward Prediction Error : Inport
  Backward Prediction Error : Inport  Port=2
  K Input : Inport  Port=3
  Delay : Delay  DelayLength=1  InitialCondition=0
  K Update Equation : Subsystem
  Sum : Sum  Inputs=|++
  Sum1 : Sum  Inputs=|++
  Forward Prediction Error Output : Outport
  Backward Prediction Error Output : Outport  Port=2
  K : Outport  Port=3
  wires:
  Sum1/1 -> Backward Prediction Error Output/1
  Delay/1 -> Sum1/2, K Update Equation/2(B I/P)
  Sum/1 -> Forward Prediction Error Output/1
  K Update Equation/2(K) -> K/1, Sum1/1
  K Update Equation/1(*K (K conjugate)) -> Sum/2
  Backward Prediction Error/1 -> Delay/1
  Forward Prediction Error/1 -> Sum/1, K Update Equation/1(F I/P)
  K Input/1 -> K Update Equation/3(K I/P)

== system FM_Bistatic_Radar_Full/Adaptive Filter/Gradiant Adaptive Lattice/50-Stage Lattice Predictor/Stage 28 ==
  note: K Update
  Forward Prediction Error : Inport
  Backward Prediction Error : Inport  Port=2
  K Input : Inport  Port=3
  Delay : Delay  DelayLength=1  InitialCondition=0
  K Update Equation : Subsystem
  Sum : Sum  Inputs=|++
  Sum1 : Sum  Inputs=|++
  Forward Prediction Error Output : Outport
  Backward Prediction Error Output : Outport  Port=2
  K : Outport  Port=3
  wires:
  Sum1/1 -> Backward Prediction Error Output/1
  Delay/1 -> Sum1/2, K Update Equation/2(B I/P)
  Sum/1 -> Forward Prediction Error Output/1
  K Update Equation/2(K) -> K/1, Sum1/1
  K Update Equation/1(*K (K conjugate)) -> Sum/2
  Backward Prediction Error/1 -> Delay/1
  Forward Prediction Error/1 -> Sum/1, K Update Equation/1(F I/P)
  K Input/1 -> K Update Equation/3(K I/P)

== system FM_Bistatic_Radar_Full/Adaptive Filter/Gradiant Adaptive Lattice/50-Stage Lattice Predictor/Stage 29 ==
  note: K Update
  Forward Prediction Error : Inport
  Backward Prediction Error : Inport  Port=2
  K Input : Inport  Port=3
  Delay : Delay  DelayLength=1  InitialCondition=0
  K Update Equation : Subsystem
  Sum : Sum  Inputs=|++
  Sum1 : Sum  Inputs=|++
  Forward Prediction Error Output : Outport
  Backward Prediction Error Output : Outport  Port=2
  K : Outport  Port=3
  wires:
  Sum1/1 -> Backward Prediction Error Output/1
  Delay/1 -> Sum1/2, K Update Equation/2(B I/P)
  Sum/1 -> Forward Prediction Error Output/1
  K Update Equation/2(K) -> K/1, Sum1/1
  K Update Equation/1(*K (K conjugate)) -> Sum/2
  Backward Prediction Error/1 -> Delay/1
  Forward Prediction Error/1 -> Sum/1, K Update Equation/1(F I/P)
  K Input/1 -> K Update Equation/3(K I/P)

== system FM_Bistatic_Radar_Full/Adaptive Filter/Gradiant Adaptive Lattice/50-Stage Lattice Predictor/Stage 3 ==
  note: K Update
  Forward Prediction Error : Inport
  Backward Prediction Error : Inport  Port=2
  K Input : Inport  Port=3
  Delay : Delay  DelayLength=1  InitialCondition=0
  K Update Equation : Subsystem
  Sum : Sum  Inputs=|++
  Sum1 : Sum  Inputs=|++
  Forward Prediction Error Output : Outport
  Backward Prediction Error Output : Outport  Port=2
  K : Outport  Port=3
  wires:
  Sum1/1 -> Backward Prediction Error Output/1
  Delay/1 -> Sum1/2, K Update Equation/2(B I/P)
  Sum/1 -> Forward Prediction Error Output/1
  K Update Equation/2(K) -> K/1, Sum1/1
  K Update Equation/1(*K (K conjugate)) -> Sum/2
  Backward Prediction Error/1 -> Delay/1
  Forward Prediction Error/1 -> Sum/1, K Update Equation/1(F I/P)
  K Input/1 -> K Update Equation/3(K I/P)

== system FM_Bistatic_Radar_Full/Adaptive Filter/Gradiant Adaptive Lattice/50-Stage Lattice Predictor/Stage 30 ==
  note: K Update
  Forward Prediction Error : Inport
  Backward Prediction Error : Inport  Port=2
  K Input : Inport  Port=3
  Delay : Delay  DelayLength=1  InitialCondition=0
  K Update Equation : Subsystem
  Sum : Sum  Inputs=|++
  Sum1 : Sum  Inputs=|++
  Forward Prediction Error Output : Outport
  Backward Prediction Error Output : Outport  Port=2
  K : Outport  Port=3
  wires:
  Sum1/1 -> Backward Prediction Error Output/1
  Delay/1 -> Sum1/2, K Update Equation/2(B I/P)
  Sum/1 -> Forward Prediction Error Output/1
  K Update Equation/2(K) -> K/1, Sum1/1
  K Update Equation/1(*K (K conjugate)) -> Sum/2
  Backward Prediction Error/1 -> Delay/1
  Forward Prediction Error/1 -> Sum/1, K Update Equation/1(F I/P)
  K Input/1 -> K Update Equation/3(K I/P)

== system FM_Bistatic_Radar_Full/Adaptive Filter/Gradiant Adaptive Lattice/50-Stage Lattice Predictor/Stage 31 ==
  note: K Update
  Forward Prediction Error : Inport
  Backward Prediction Error : Inport  Port=2
  K Input : Inport  Port=3
  Delay : Delay  DelayLength=1  InitialCondition=0
  K Update Equation : Subsystem
  Sum : Sum  Inputs=|++
  Sum1 : Sum  Inputs=|++
  Forward Prediction Error Output : Outport
  Backward Prediction Error Output : Outport  Port=2
  K : Outport  Port=3
  wires:
  Sum1/1 -> Backward Prediction Error Output/1
  Delay/1 -> Sum1/2, K Update Equation/2(B I/P)
  Sum/1 -> Forward Prediction Error Output/1
  K Update Equation/2(K) -> K/1, Sum1/1
  K Update Equation/1(*K (K conjugate)) -> Sum/2
  Backward Prediction Error/1 -> Delay/1
  Forward Prediction Error/1 -> Sum/1, K Update Equation/1(F I/P)
  K Input/1 -> K Update Equation/3(K I/P)

== system FM_Bistatic_Radar_Full/Adaptive Filter/Gradiant Adaptive Lattice/50-Stage Lattice Predictor/Stage 32 ==
  note: K Update
  Forward Prediction Error : Inport
  Backward Prediction Error : Inport  Port=2
  K Input : Inport  Port=3
  Delay : Delay  DelayLength=1  InitialCondition=0
  K Update Equation : Subsystem
  Sum : Sum  Inputs=|++
  Sum1 : Sum  Inputs=|++
  Forward Prediction Error Output : Outport
  Backward Prediction Error Output : Outport  Port=2
  K : Outport  Port=3
  wires:
  Sum1/1 -> Backward Prediction Error Output/1
  Delay/1 -> Sum1/2, K Update Equation/2(B I/P)
  Sum/1 -> Forward Prediction Error Output/1
  K Update Equation/2(K) -> K/1, Sum1/1
  K Update Equation/1(*K (K conjugate)) -> Sum/2
  Backward Prediction Error/1 -> Delay/1
  Forward Prediction Error/1 -> Sum/1, K Update Equation/1(F I/P)
  K Input/1 -> K Update Equation/3(K I/P)

== system FM_Bistatic_Radar_Full/Adaptive Filter/Gradiant Adaptive Lattice/50-Stage Lattice Predictor/Stage 33 ==
  note: K Update
  Forward Prediction Error : Inport
  Backward Prediction Error : Inport  Port=2
  K Input : Inport  Port=3
  Delay : Delay  DelayLength=1  InitialCondition=0
  K Update Equation : Subsystem
  Sum : Sum  Inputs=|++
  Sum1 : Sum  Inputs=|++
  Forward Prediction Error Output : Outport
  Backward Prediction Error Output : Outport  Port=2
  K : Outport  Port=3
  wires:
  Sum1/1 -> Backward Prediction Error Output/1
  Delay/1 -> Sum1/2, K Update Equation/2(B I/P)
  Sum/1 -> Forward Prediction Error Output/1
  K Update Equation/2(K) -> K/1, Sum1/1
  K Update Equation/1(*K (K conjugate)) -> Sum/2
  Backward Prediction Error/1 -> Delay/1
  Forward Prediction Error/1 -> Sum/1, K Update Equation/1(F I/P)
  K Input/1 -> K Update Equation/3(K I/P)

== system FM_Bistatic_Radar_Full/Adaptive Filter/Gradiant Adaptive Lattice/50-Stage Lattice Predictor/Stage 34 ==
  note: K Update
  Forward Prediction Error : Inport
  Backward Prediction Error : Inport  Port=2
  K Input : Inport  Port=3
  Delay : Delay  DelayLength=1  InitialCondition=0
  K Update Equation : Subsystem
  Sum : Sum  Inputs=|++
  Sum1 : Sum  Inputs=|++
  Forward Prediction Error Output : Outport
  Backward Prediction Error Output : Outport  Port=2
  K : Outport  Port=3
  wires:
  Sum1/1 -> Backward Prediction Error Output/1
  Delay/1 -> Sum1/2, K Update Equation/2(B I/P)
  Sum/1 -> Forward Prediction Error Output/1
  K Update Equation/2(K) -> K/1, Sum1/1
  K Update Equation/1(*K (K conjugate)) -> Sum/2
  Backward Prediction Error/1 -> Delay/1
  Forward Prediction Error/1 -> Sum/1, K Update Equation/1(F I/P)
  K Input/1 -> K Update Equation/3(K I/P)

== system FM_Bistatic_Radar_Full/Adaptive Filter/Gradiant Adaptive Lattice/50-Stage Lattice Predictor/Stage 35 ==
  note: K Update
  Forward Prediction Error : Inport
  Backward Prediction Error : Inport  Port=2
  K Input : Inport  Port=3
  Delay : Delay  DelayLength=1  InitialCondition=0
  K Update Equation : Subsystem
  Sum : Sum  Inputs=|++
  Sum1 : Sum  Inputs=|++
  Forward Prediction Error Output : Outport
  Backward Prediction Error Output : Outport  Port=2
  K : Outport  Port=3
  wires:
  Sum1/1 -> Backward Prediction Error Output/1
  Delay/1 -> Sum1/2, K Update Equation/2(B I/P)
  Sum/1 -> Forward Prediction Error Output/1
  K Update Equation/2(K) -> K/1, Sum1/1
  K Update Equation/1(*K (K conjugate)) -> Sum/2
  Backward Prediction Error/1 -> Delay/1
  Forward Prediction Error/1 -> Sum/1, K Update Equation/1(F I/P)
  K Input/1 -> K Update Equation/3(K I/P)

== system FM_Bistatic_Radar_Full/Adaptive Filter/Gradiant Adaptive Lattice/50-Stage Lattice Predictor/Stage 36 ==
  note: K Update
  Forward Prediction Error : Inport
  Backward Prediction Error : Inport  Port=2
  K Input : Inport  Port=3
  Delay : Delay  DelayLength=1  InitialCondition=0
  K Update Equation : Subsystem
  Sum : Sum  Inputs=|++
  Sum1 : Sum  Inputs=|++
  Forward Prediction Error Output : Outport
  Backward Prediction Error Output : Outport  Port=2
  K : Outport  Port=3
  wires:
  Sum1/1 -> Backward Prediction Error Output/1
  Delay/1 -> Sum1/2, K Update Equation/2(B I/P)
  Sum/1 -> Forward Prediction Error Output/1
  K Update Equation/2(K) -> K/1, Sum1/1
  K Update Equation/1(*K (K conjugate)) -> Sum/2
  Backward Prediction Error/1 -> Delay/1
  Forward Prediction Error/1 -> Sum/1, K Update Equation/1(F I/P)
  K Input/1 -> K Update Equation/3(K I/P)

== system FM_Bistatic_Radar_Full/Adaptive Filter/Gradiant Adaptive Lattice/50-Stage Lattice Predictor/Stage 37 ==
  note: K Update
  Forward Prediction Error : Inport
  Backward Prediction Error : Inport  Port=2
  K Input : Inport  Port=3
  Delay : Delay  DelayLength=1  InitialCondition=0
  K Update Equation : Subsystem
  Sum : Sum  Inputs=|++
  Sum1 : Sum  Inputs=|++
  Forward Prediction Error Output : Outport
  Backward Prediction Error Output : Outport  Port=2
  K : Outport  Port=3
  wires:
  Sum1/1 -> Backward Prediction Error Output/1
  Delay/1 -> Sum1/2, K Update Equation/2(B I/P)
  Sum/1 -> Forward Prediction Error Output/1
  K Update Equation/2(K) -> K/1, Sum1/1
  K Update Equation/1(*K (K conjugate)) -> Sum/2
  Backward Prediction Error/1 -> Delay/1
  Forward Prediction Error/1 -> Sum/1, K Update Equation/1(F I/P)
  K Input/1 -> K Update Equation/3(K I/P)

== system FM_Bistatic_Radar_Full/Adaptive Filter/Gradiant Adaptive Lattice/50-Stage Lattice Predictor/Stage 38 ==
  note: K Update
  Forward Prediction Error : Inport
  Backward Prediction Error : Inport  Port=2
  K Input : Inport  Port=3
  Delay : Delay  DelayLength=1  InitialCondition=0
  K Update Equation : Subsystem
  Sum : Sum  Inputs=|++
  Sum1 : Sum  Inputs=|++
  Forward Prediction Error Output : Outport
  Backward Prediction Error Output : Outport  Port=2
  K : Outport  Port=3
  wires:
  Sum1/1 -> Backward Prediction Error Output/1
  Delay/1 -> Sum1/2, K Update Equation/2(B I/P)
  Sum/1 -> Forward Prediction Error Output/1
  K Update Equation/2(K) -> K/1, Sum1/1
  K Update Equation/1(*K (K conjugate)) -> Sum/2
  Backward Prediction Error/1 -> Delay/1
  Forward Prediction Error/1 -> Sum/1, K Update Equation/1(F I/P)
  K Input/1 -> K Update Equation/3(K I/P)

== system FM_Bistatic_Radar_Full/Adaptive Filter/Gradiant Adaptive Lattice/50-Stage Lattice Predictor/Stage 39 ==
  note: K Update
  Forward Prediction Error : Inport
  Backward Prediction Error : Inport  Port=2
  K Input : Inport  Port=3
  Delay : Delay  DelayLength=1  InitialCondition=0
  K Update Equation : Subsystem
  Sum : Sum  Inputs=|++
  Sum1 : Sum  Inputs=|++
  Forward Prediction Error Output : Outport
  Backward Prediction Error Output : Outport  Port=2
  K : Outport  Port=3
  wires:
  Sum1/1 -> Backward Prediction Error Output/1
  Delay/1 -> Sum1/2, K Update Equation/2(B I/P)
  Sum/1 -> Forward Prediction Error Output/1
  K Update Equation/2(K) -> K/1, Sum1/1
  K Update Equation/1(*K (K conjugate)) -> Sum/2
  Backward Prediction Error/1 -> Delay/1
  Forward Prediction Error/1 -> Sum/1, K Update Equation/1(F I/P)
  K Input/1 -> K Update Equation/3(K I/P)

== system FM_Bistatic_Radar_Full/Adaptive Filter/Gradiant Adaptive Lattice/50-Stage Lattice Predictor/Stage 4 ==
  note: K Update
  Forward Prediction Error : Inport
  Backward Prediction Error : Inport  Port=2
  K Input : Inport  Port=3
  Delay : Delay  DelayLength=1  InitialCondition=0
  K Update Equation : Subsystem
  Sum : Sum  Inputs=|++
  Sum1 : Sum  Inputs=|++
  Forward Prediction Error Output : Outport
  Backward Prediction Error Output : Outport  Port=2
  K : Outport  Port=3
  wires:
  Sum1/1 -> Backward Prediction Error Output/1
  Delay/1 -> Sum1/2, K Update Equation/2(B I/P)
  Sum/1 -> Forward Prediction Error Output/1
  K Update Equation/2(K) -> K/1, Sum1/1
  K Update Equation/1(*K (K conjugate)) -> Sum/2
  Backward Prediction Error/1 -> Delay/1
  Forward Prediction Error/1 -> Sum/1, K Update Equation/1(F I/P)
  K Input/1 -> K Update Equation/3(K I/P)

== system FM_Bistatic_Radar_Full/Adaptive Filter/Gradiant Adaptive Lattice/50-Stage Lattice Predictor/Stage 40 ==
  note: K Update
  Forward Prediction Error : Inport
  Backward Prediction Error : Inport  Port=2
  K Input : Inport  Port=3
  Delay : Delay  DelayLength=1  InitialCondition=0
  K Update Equation : Subsystem
  Sum : Sum  Inputs=|++
  Sum1 : Sum  Inputs=|++
  Forward Prediction Error Output : Outport
  Backward Prediction Error Output : Outport  Port=2
  K : Outport  Port=3
  wires:
  Sum1/1 -> Backward Prediction Error Output/1
  Delay/1 -> Sum1/2, K Update Equation/2(B I/P)
  Sum/1 -> Forward Prediction Error Output/1
  K Update Equation/2(K) -> K/1, Sum1/1
  K Update Equation/1(*K (K conjugate)) -> Sum/2
  Backward Prediction Error/1 -> Delay/1
  Forward Prediction Error/1 -> Sum/1, K Update Equation/1(F I/P)
  K Input/1 -> K Update Equation/3(K I/P)
